simulink model "Main_v2"  (R2022b)
settings: Solver=ode23  StartTime=0.0  StopTime=sim_time-0.02
values from neighbouring files (symbols this model uses):
  bike_model = 1    [Main_sim.m]    (also in Startup_Script.m; Startup_Script_v2.m)
  bike_params = LoadBikeParameters(bike)    [Kalman_offline.m]    (also in Main_sim.m; Startup_Script.m; Startup_Script_v2.m; Startup_labview.m)
  C1 = [1 0 0 0 0 0 0 ... (first row only)    [Kalman_offline.m]    (also in Main_sim.m; Startup_Script.m; Startup_Script_v2.m; Startup_labview.m)
  counter = (Ts_GPS / Ts) - 1    (= 9)    [Kalman_offline.m]    (also in Main_sim.m; Startup_Script.m; Startup_Script_v2.m; Startup_labview.m)
  D_balancing_inner = 0    [Main_sim.m]    (also in Startup_Script.m; Startup_Script_v2.m; Startup_labview.m)
  D_balancing_outer = 0.0    (= 0)    [Main_sim.m]    (also in Startup_Script.m; Startup_Script_v2.m; Startup_labview.m)
  e1_max = abs(-k2*e2_max/k1)    [Main_sim.m]    (also in Startup_Script.m; Startup_Script_v2.m; Startup_labview.m)
  g = -9.81    [Kalman_offline.m]    (also in Main_sim.m = 9.81; Startup_Script.m = 9.81; Startup_Script_v2.m = 9.81; Startup_labview.m = 9.81)
  hor_dis = 10    [Main_sim.m]    (also in Startup_Script.m = 1; Startup_Script_v2.m = 1)
  I_balancing_inner = 0    [Main_sim.m]    (also in Startup_Script.m; Startup_Script_v2.m; Startup_labview.m)
  I_balancing_outer = 0.0    (= 0)    [Main_sim.m]    (also in Startup_Script.m; Startup_Script_v2.m; Startup_labview.m)
  initial_state_estimate = initial_state    [Main_sim.m]    (also in Startup_Script.m; Startup_Script_v2.m)
  k1 = K(1)    [Main_sim.m]    (also in Startup_Script.m; Startup_Script_v2.m; Startup_labview.m)
  k2 = K(2)    [Main_sim.m]    (also in Startup_Script.m; Startup_Script_v2.m; Startup_labview.m)
  Kalman_gain1 = Kalman_gain1'    [Kalman_offline.m]    (also in Main_sim.m; Startup_Script.m; Startup_Script_v2.m; Startup_labview.m)
  Kalman_gain2 = Kalman_gain2'    [Kalman_offline.m]    (also in Main_sim.m = Kalman_gain1(4:7,3:7); Startup_Script.m; Startup_Script_v2.m; Startup_labview.m = Kalman_gain1(4:7,3:7))
  linearized_sys = ss(A,B,C,D)    [Startup_Script_v2.m]
  P_balancing_inner = 3    [Main_sim.m]    (also in Startup_Script.m; Startup_Script_v2.m; Startup_labview.m = 1)
  P_balancing_outer = 1.3    [Main_sim.m]    (also in Startup_Script.m; Startup_Script_v2.m; Startup_labview.m = 1.75)
  Psiref = psiref'    [ReferenceGenerator.m]
  ref_dis = 0.01    [Main_sim.m]    (also in Startup_Script.m; Startup_Script_v2.m)
  ref_start_idx = 2    [Main_sim.m]    (also in Startup_Script.m; Startup_Script_v2.m)
  Ts = 0.01    [Kalman_offline.m]    (also in Main_sim.m; Startup_Script.m; Startup_Script_v2.m; Startup_labview.m)
  v = 3    [Main_sim.m]    (also in Startup_Script.m; Startup_Script_v2.m; Startup_labview.m = 2; Test_ss.m)
  Xref = xref'    [ReferenceGenerator.m]
  Yref = yref'    [ReferenceGenerator.m]
undefined symbols (not defined in the file or in its folder): initial_state, pert_deltadot_state, pert_deltadot_state_fun, pert_phidot_state, pert_phidot_state_fun
libraries: eeGeneralControl x3, slpidlib x2, simulink x2, cstblocks x1
(part 1 of 2)
settings Model: PauseTimes=0.16  Creator=Hadi Hajieghrary  LastModifiedBy=levi1
settings SolverCC: MaxConsecutiveMinStep=10  ZeroCrossAlgorithm=Adaptive  AlgebraicLoopSolver=TrustRegion  AutoInsertRateTranBlk=on
settings DebuggingCC: AlgebraicLoopMsg=none  UnconnectedInputMsg=warning  UnconnectedOutputMsg=warning  UnconnectedLineMsg=warning
settings ModelReferenceCC: EnableRefExpFcnMdlSchedulingChecks=on
settings RTWCC: DLArmComputeVersion=19.05

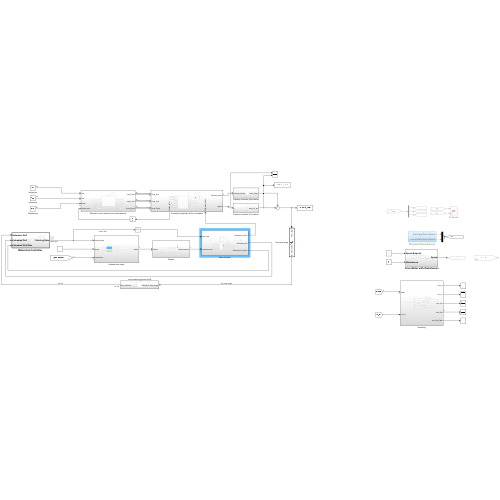
[thumbnail: Simulink's stored preview of the top-level diagram]
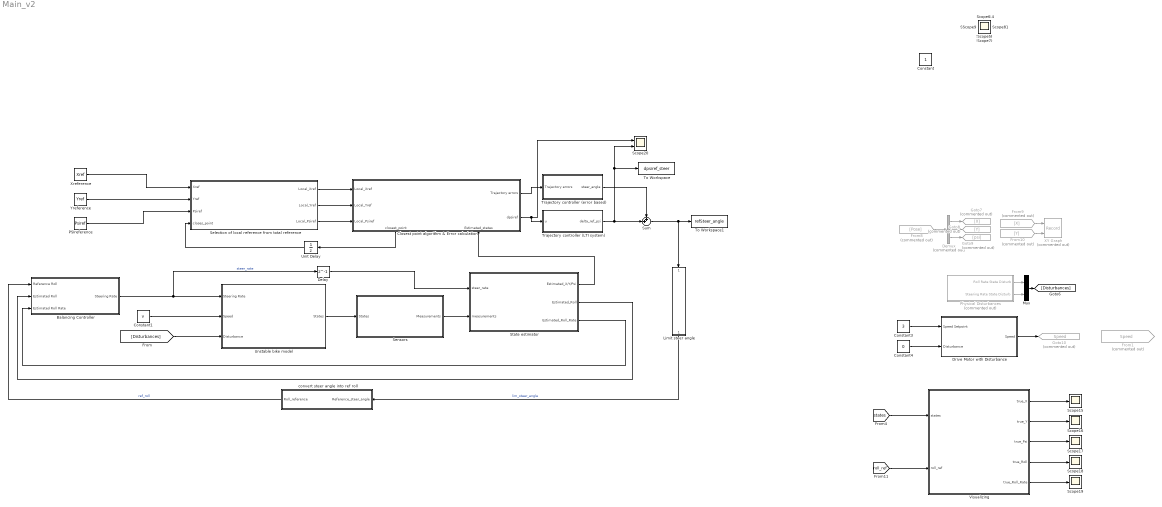
== system Main_v2 ==
  "Balancing Controller " : Subsystem  TreatAsAtomicUnit=on  SystemSampleTime=Ts
      settings: MinAlgLoopOccurrences=on
  Closest point algorithm & Error calculation : Subsystem
      settings: PortSchema="{\"entries\":[{\"content\":{\"sides\":[{\"content\":{\"connectorIds\":[\"In1\",\"In2\",\"In3\"]},\"type\":\"ConnectorPlacement.EquallySpacedRectSide\",\"uuid\":\"cc846df4-97c1-4e38-a551-63d96742d514\"},{\"content\":{\"connectorIds\":[\"Out1\",\"Out2\"],\"side\":\"RIGHT\"},\"type\":\"ConnectorPlacement.EquallySpacedRectSide\",\"uuid\":\"926eeee4-c51a-40d9-a9a1-df7a0c76cd55\"},{\"content\":{\"connectorIds\":[],\"side\":\"TOP\"},\"type\":\"ConnectorPlacement.EquallySpacedRectSide\",\"uuid\":\"e902e63c-5309-44b2-99e1-76b44c06d1f2\"},{\"content\":{\"connectorIds\":[\"Out3\",\"In4\"],\"side\":\"BOTTOM\"},\"type\":\"ConnectorPlacement.EquallySpacedRectSide\",\"uuid\":\"f92d60b4-b11f-4907-83c4-1907c5b6c496\"}]},\"type\":\"ConnectorPlacement.EquallySpacedConnector\",\"uuid\":\"17b67b4e-0a47-44a6-bf11-0cf8a9b1982c\"}],\"packageUris\":[\"http://schema.mathworks.com/mf0/Connector/R2020b\"],\"version\":\"1.0\"}"
  Constant1 : Constant  Value=v
  Constant3 : Constant  Value=3
  Constant4 : Constant  Value=0
  Delay : Delay  DelayLength=1  SampleTime=Ts
  Demux : Demux  Commented=on  Outputs=3
  Drive Motor with Disturbance : Subsystem
  From1 : From  Commented=on  GotoTag=Speed  TagVisibility=global
  From10 : From  Commented=on  GotoTag=Y
  From8 : From  Commented=on  GotoTag=Pose
  From9 : From  Commented=on  GotoTag=X
  Goto10 : Goto  Commented=on  GotoTag=Speed  TagVisibility=global
  Goto7 : Goto  Commented=on  GotoTag=X
  Goto8 : Goto  Commented=on  GotoTag=Y
  Goto9 : Goto  Commented=on  GotoTag=psi
  Limit steer angle : MATLAB Function  TreatAsAtomicUnit=on
  Mux : Mux  Inputs=2
  PSIreference : Constant  Value=Psiref
  Physical Disturbances : Subsystem  Commented=on
  Scope{,1..19} (20 alike) : Scope
  Scope20 : Scope  NumInputPorts=2
  Selection of local reference from total reference : Subsystem
  Sensors : Subsystem
  State estimator : Subsystem
  Sum : Sum  Inputs=++|
  To Workspace : ToWorkspace  VariableName=dpsiref_steer  SaveFormat=Timeseries  SampleTime=-1
  To Workspace1 : ToWorkspace  VariableName=refSteer_angle  SaveFormat=Timeseries  SampleTime=-1
  Trajectory controller (LTI system) : Subsystem
  Trajectory controller (error based) : Subsystem
  Unit Delay : UnitDelay  InitialCondition=ref_start_idx  SampleTime=Ts  HasFrameUpgradeWarning=on
  Unstable bike model : Subsystem
  Visualizing : Subsystem
  XY Graph : Record  Commented=on  FileSettingsInternal="{\"entries\":[{\"content\":{\"excelSettings\":{\"content\":{},\"type\":\"Streamout.ExcelSettings\"}},\"type\":\"Streamout.FileSettingStorage\",\"uuid\":\"82b19030-816e-4949-ae29-c4c1f1632771\"}],\"packageUris\":[\"http://schema.mathworks.com/mf0/streamout_blocks/R2020a\"],\"version\":\"1.0\"}"  Layout=[1 1]  SignalsInternal="{\"entries\":[{\"content\":{\"signals\":[]},\"type\":\"RecordBlkView.InputSignals\",\"uuid\":\"cc5346bf-f4f9-4ee2-bd9b-070395d24a3d\"}],\"packageUris\":[\"http://schema.mathworks.com/mf0/streamout_blocks/R2020a\"],\"version\":\"1.0\"}"  VisualizationBindings="{\"xyplotplugin\":{\"info\":[{\"series\":[],\"subplotID\":1}]}}"  CompatibilityTag=XY
  Xreference : Constant  Value=Xref
  Yreference : Constant  Value=Yref
  convert steer angle into ref roll : Subsystem
  Constant : Constant  IOType=siggen
  wires:
  From8/1 -> Demux/1
  Demux/1 -> Goto7/1
  Demux/2 -> Goto8/1
  Demux/3 -> Goto9/1
  From10/1 -> XY Graph/2
  From9/1 -> XY Graph/1
  Physical Disturbances/1(Roll Rate State Disturb) -> Mux/1
  Physical Disturbances/2(Steering Rate State Disturb) -> Mux/2
  Mux/1 -> [Disturbances]
  Drive Motor with Disturbance/1(Speed) -> Goto10/1
  Constant3/1 -> Drive Motor with Disturbance/1(Speed Setpoint)
  Constant4/1 -> Drive Motor with Disturbance/2(Disturbance)
  "Balancing Controller "/1(Steering Rate) -> Delay/1, Unstable bike model/1(Steering Rate)  "steer_rate"
  Selection of local reference from total reference/1(Local_Xref) -> Closest point algorithm & Error calculation/1(Local_Xref)
  Closest point algorithm & Error calculation/3(closest_point) -> Unit Delay/1
  Unit Delay/1 -> Selection of local reference from total reference/4(closes_point)
  Trajectory controller (error based)/1(steer_angle) -> Sum/1
  Closest point algorithm & Error calculation/2(dpsiref) -> Trajectory controller (LTI system)/1(u), Scope20/1
  Sum/1 -> Limit steer angle/1(steer_angle), To Workspace1/1
  Limit steer angle/1(lim_steer_angle) -> convert steer angle into ref roll/1(Reference_steer_angle)  "lim_steer_angle"
  convert steer angle into ref roll/1(Roll_reference) -> "Balancing Controller "/1(Reference Roll)  "ref_roll"
  [Disturbances] -> Unstable bike model/3(Disturbance)
  Sensors/1(Measurements) -> State estimator/2(measurements)
  Selection of local reference from total reference/2(Local_Yref) -> Closest point algorithm & Error calculation/2(Local_Yref)
  Selection of local reference from total reference/3(Local_Psiref) -> Closest point algorithm & Error calculation/3(Local_Psiref)
  [states] -> Visualizing/1(states)
  Visualizing/1(true_X) -> Scope15/1
  Visualizing/2(true_Y) -> Scope16/1
  Visualizing/3(true_Psi) -> Scope17/1
  Visualizing/4(true_Roll) -> Scope18/1
  Visualizing/5(true_Roll_Rate) -> Scope19/1
  [roll_ref] -> Visualizing/2(roll_ref)
  Unstable bike model/1(States) -> Sensors/1(States)
  Constant1/1 -> Unstable bike model/2(Speed)
  State estimator/2(Estimated_Roll) -> "Balancing Controller "/2(Estimated Roll)
  State estimator/3(Estimated_Roll_Rate) -> "Balancing Controller "/3(Estimated Roll Rate)
  Xreference/1 -> Selection of local reference from total reference/1(Xref)
  Yreference/1 -> Selection of local reference from total reference/2(Yref)
  PSIreference/1 -> Selection of local reference from total reference/3(Psiref)
  Delay/1 -> State estimator/1(steer_rate)
  State estimator/1(Estimated_X/Y/Psi) -> Closest point algorithm & Error calculation/4(Estimated_states)
  Closest point algorithm & Error calculation/1(Trajectory errors) -> Trajectory controller (error based)/1(Trajectory errors)
  Trajectory controller (LTI system)/1(delta_ref_psi) -> To Workspace/1, Scope20/2, Sum/2

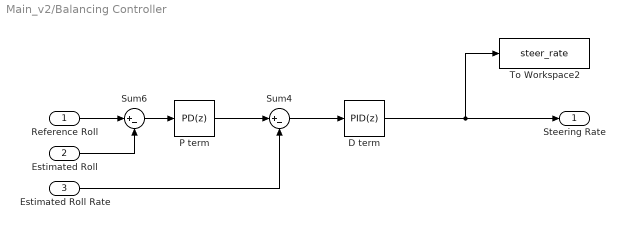
== system Main_v2/Balancing Controller  ==
  Reference Roll : Inport
  Estimated Roll : Inport  Port=2
  Estimated Roll Rate : Inport  Port=3
  D term : slpidlib/PID Controller  Controller=PID  Form=Parallel  TimeDomain=Discrete-time  UseExternalTs=off  SampleTime=Ts  IntegratorMethod=Forward Euler  FilterMethod=Forward Euler  ControllerParametersSource=internal  P=P_balancing_inner  I=I_balancing_inner  UseKiTs=off  D=D_balancing_inner  N=100  UseFilter=off  TunerSelectOption=Transfer Function Based (PID Tuner App)  InitialConditionSource=internal  InitialConditionForIntegrator=0  InitialConditionForFilter=0  DifferentiatorICPrevScaledInput=0  ExternalReset=none  TrackingMode=off  Kt=1  LimitOutput=off  SatLimitsSource=internal  UpperSaturationLimit=inf  LowerSaturationLimit=-inf  LinearizeAsGain=on  AntiWindupMode=none  Kb=1  LimitIntegrator=off  UpperIntegratorSaturationLimit=inf  LowerIntegratorSaturationLimit=-inf  POutMin=[]  POutMax=[]  IOutMin=[]  IOutMax=[]  DOutMin=[]  DOutMax=[]  NOutMin=[]  NOutMax=[]  SumOutMin=[]  SumOutMax=[]  SaturationOutMin=[]  SaturationOutMax=[]  PParamMin=[]  PParamMax=[]  IParamMin=[]  IParamMax=[]  DParamMin=[]  DParamMax=[]  NParamMin=[]  NParamMax=[]  KbParamMin=[]  KbParamMax=[]  KtParamMin=[]  KtParamMax=[]  KbOutMin=[]  KbOutMax=[]  KtOutMin=[]  KtOutMax=[]  IntegratorOutMin=[]  IntegratorOutMax=[]  FilterOutMin=[]  FilterOutMax=[]  SumI1OutMin=[]  SumI1OutMax=[]  SumI2OutMin=[]  SumI2OutMax=[]  SumI3OutMin=[]  SumI3OutMax=[]  SumI4OutMin=[]  SumI4OutMax=[]  SumDOutMin=[]  SumDOutMax=[]  DifferentiatorOutMin=[]  DifferentiatorOutMax=[]  FilterDiffOutCoefMin=[]  FilterDiffOutCoefMax=[]  ReciprocalOutMin=[]  ReciprocalOutMax=[]  SumDenOutMin=[]  SumDenOutMax=[]  SumNumOutMin=[]  SumNumOutMax=[]  DivideOutMin=[]  DivideOutMax=[]  UdiffTsProdOutMin=[]  UdiffTsProdOutMax=[]  NTsProdOutMin=[]  NTsProdOutMax=[]  UintegralTsProdOutMin=[]  UintegralTsProdOutMax=[]  UngainTsProdOutMin=[]  UngainTsProdOutMax=[]  IntegratorContinuousStateAttributes=''  IntegratorStateMustResolveToSignalObject=off  IntegratorRTWStateStorageClass=Auto  FilterContinuousStateAttributes=''  FilterStateMustResolveToSignalObject=off  FilterRTWStateStorageClass=Auto  ParallelPVariant=InternalParameters  IdealPVariant=Disabled  IVariant=InternalParameters  DVariant=InternalParameters  IntegratorVariant=Discrete  SatVariant=Disabled  AWVariant=Passthrough  PCopyVariant=Disabled  TRVariant=Disabled  FdbkBlocksVariant=Forward  IdealPFdbkVariant=Disabled  SatFdbkVariant=Disabled  DerivativeFilterVariant=Differentiator  NVariant=Passthrough  NCopyVariant=Disabled_SignalSpec  FilterICVariant=InternalICsDifferentiator  IntegratorICVariant=InternalICs  ExternalResetVariant=Disabled  TRSumVariant=Passthrough  SumFdbkVariant=Disabled  SumVariant=Sum_PID  TsampFilterVariant=InternalTs  TsampNgainVariant=Passthrough  TsampIntegralVariant=Passthrough  ExternalSaturationOutDataTypeStr=Inherit: Same as second input
  P term : slpidlib/PID Controller  Controller=PD  Form=Parallel  TimeDomain=Discrete-time  UseExternalTs=off  SampleTime=Ts  IntegratorMethod=Forward Euler  FilterMethod=Forward Euler  ControllerParametersSource=internal  P=P_balancing_outer  I=I_balancing_outer  UseKiTs=off  D=D_balancing_outer  N=100  UseFilter=off  TunerSelectOption=Transfer Function Based (PID Tuner App)  InitialConditionSource=internal  InitialConditionForIntegrator=0  InitialConditionForFilter=0  DifferentiatorICPrevScaledInput=0  ExternalReset=none  TrackingMode=off  Kt=1  LimitOutput=off  SatLimitsSource=internal  UpperSaturationLimit=inf  LowerSaturationLimit=-inf  LinearizeAsGain=on  AntiWindupMode=none  Kb=1  LimitIntegrator=off  UpperIntegratorSaturationLimit=inf  LowerIntegratorSaturationLimit=-inf  POutMin=[]  POutMax=[]  IOutMin=[]  IOutMax=[]  DOutMin=[]  DOutMax=[]  NOutMin=[]  NOutMax=[]  SumOutMin=[]  SumOutMax=[]  SaturationOutMin=[]  SaturationOutMax=[]  PParamMin=[]  PParamMax=[]  IParamMin=[]  IParamMax=[]  DParamMin=[]  DParamMax=[]  NParamMin=[]  NParamMax=[]  KbParamMin=[]  KbParamMax=[]  KtParamMin=[]  KtParamMax=[]  KbOutMin=[]  KbOutMax=[]  KtOutMin=[]  KtOutMax=[]  IntegratorOutMin=[]  IntegratorOutMax=[]  FilterOutMin=[]  FilterOutMax=[]  SumI1OutMin=[]  SumI1OutMax=[]  SumI2OutMin=[]  SumI2OutMax=[]  SumI3OutMin=[]  SumI3OutMax=[]  SumI4OutMin=[]  SumI4OutMax=[]  SumDOutMin=[]  SumDOutMax=[]  DifferentiatorOutMin=[]  DifferentiatorOutMax=[]  FilterDiffOutCoefMin=[]  FilterDiffOutCoefMax=[]  ReciprocalOutMin=[]  ReciprocalOutMax=[]  SumDenOutMin=[]  SumDenOutMax=[]  SumNumOutMin=[]  SumNumOutMax=[]  DivideOutMin=[]  DivideOutMax=[]  UdiffTsProdOutMin=[]  UdiffTsProdOutMax=[]  NTsProdOutMin=[]  NTsProdOutMax=[]  UintegralTsProdOutMin=[]  UintegralTsProdOutMax=[]  UngainTsProdOutMin=[]  UngainTsProdOutMax=[]  IntegratorContinuousStateAttributes=''  IntegratorStateMustResolveToSignalObject=off  IntegratorRTWStateStorageClass=Auto  FilterContinuousStateAttributes=''  FilterStateMustResolveToSignalObject=off  FilterRTWStateStorageClass=Auto  ParallelPVariant=InternalParameters  IdealPVariant=Disabled  IVariant=Disabled  DVariant=InternalParameters  IntegratorVariant=Disabled  SatVariant=Disabled  AWVariant=Disabled  PCopyVariant=Disabled  TRVariant=Disabled  FdbkBlocksVariant=Forward  IdealPFdbkVariant=Disabled  SatFdbkVariant=Disabled  DerivativeFilterVariant=Differentiator  NVariant=Passthrough  NCopyVariant=Disabled_SignalSpec  FilterICVariant=InternalICsDifferentiator  IntegratorICVariant=Disabled  ExternalResetVariant=Disabled  TRSumVariant=Passthrough  SumFdbkVariant=Disabled  SumVariant=Sum_PD  TsampFilterVariant=InternalTs  TsampNgainVariant=Passthrough  TsampIntegralVariant=Disabled_SignalSpec  ExternalSaturationOutDataTypeStr=Inherit: Same as second input
  Sum4 : Sum  Inputs=|+-
  Sum6 : Sum  Inputs=|+-
  To Workspace2 : ToWorkspace  VariableName=steer_rate  SaveFormat=Timeseries  SampleTime=-1
  Steering Rate : Outport
  wires:
  Sum4/1 -> D term/1
  Reference Roll/1 -> Sum6/1
  Sum6/1 -> P term/1
  Estimated Roll Rate/1 -> Sum4/2
  P term/1 -> Sum4/1
  D term/1 -> To Workspace2/1, Steering Rate/1
  Estimated Roll/1 -> Sum6/2

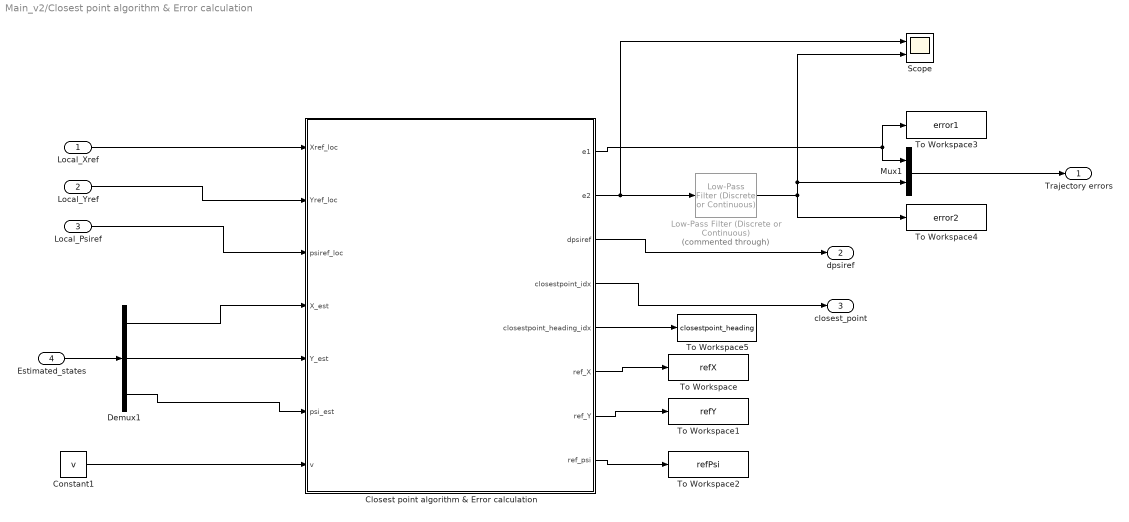
== system Main_v2/Closest point algorithm & Error calculation ==
  Local_Xref : Inport
  Local_Yref : Inport  Port=2
  Local_Psiref : Inport  Port=3
  Estimated_states : Inport  Port=4
  Closest point algorithm & Error calculation : MATLAB Function  TreatAsAtomicUnit=on
  Constant1 : Constant  Value=v
  Demux1 : Demux  Outputs=3
  Low-Pass Filter (Discrete or Continuous) : eeGeneralControl/Low-Pass Filter (Discrete or Continuous)  Commented=through  K=1  T=1  B=inf  A=-inf  init_option=Inherited from block input  x0=0  Ts=Ts
  Mux1 : Mux  Inputs=2
  Scope : Scope  NumInputPorts=2
  To Workspace : ToWorkspace  VariableName=refX  SaveFormat=Timeseries  SampleTime=-1
  To Workspace1 : ToWorkspace  VariableName=refY  SaveFormat=Timeseries  SampleTime=-1
  To Workspace2 : ToWorkspace  VariableName=refPsi  SaveFormat=Timeseries  SampleTime=-1
  To Workspace3 : ToWorkspace  VariableName=error1  SaveFormat=Timeseries  SampleTime=-1
  To Workspace4 : ToWorkspace  VariableName=error2  SaveFormat=Timeseries  SampleTime=-1
  To Workspace5 : ToWorkspace  VariableName=closestpoint_heading  SaveFormat=Timeseries  SampleTime=-1
  Trajectory errors : Outport
  dpsiref : Outport  Port=2
  closest_point : Outport  Port=3
  wires:
  Closest point algorithm & Error calculation/7(ref_Y) -> To Workspace1/1
  Constant1/1 -> Closest point algorithm & Error calculation/7(v)
  Closest point algorithm & Error calculation/8(ref_psi) -> To Workspace2/1
  Closest point algorithm & Error calculation/3(dpsiref) -> dpsiref/1
  Closest point algorithm & Error calculation/4(closestpoint_idx) -> closest_point/1
  Closest point algorithm & Error calculation/6(ref_X) -> To Workspace/1
  Demux1/2 -> Closest point algorithm & Error calculation/5(Y_est)
  Demux1/1 -> Closest point algorithm & Error calculation/4(X_est)
  Estimated_states/1 -> Demux1/1
  Local_Psiref/1 -> Closest point algorithm & Error calculation/3(psiref_loc)
  Local_Yref/1 -> Closest point algorithm & Error calculation/2(Yref_loc)
  Local_Xref/1 -> Closest point algorithm & Error calculation/1(Xref_loc)
  Closest point algorithm & Error calculation/1(e1) -> To Workspace3/1, Mux1/1
  Closest point algorithm & Error calculation/2(e2) -> Scope/1, Low-Pass Filter (Discrete or Continuous)/1
  Mux1/1 -> Trajectory errors/1
  Closest point algorithm & Error calculation/5(closestpoint_heading_idx) -> To Workspace5/1
  Low-Pass Filter (Discrete or Continuous)/1 -> Mux1/2, Scope/2, To Workspace4/1
  Demux1/3 -> Closest point algorithm & Error calculation/6(psi_est)

== system Main_v2/Drive Motor with Disturbance ==
  Speed Setpoint : Inport
  Disturbance : Inport  Port=2
  Sum2 : Sum  Inputs=++|
  Transfer Fcn : TransferFcn  Denominator=[2 1]
  Speed : Outport
  wires:
  Sum2/1 -> Speed/1
  Transfer Fcn/1 -> Sum2/2
  Speed Setpoint/1 -> Transfer Fcn/1
  Disturbance/1 -> Sum2/1

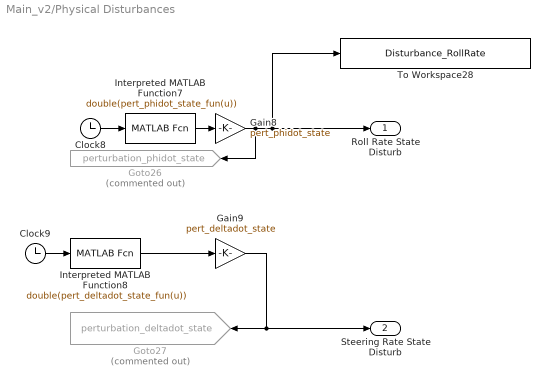
== system Main_v2/Physical Disturbances ==
  Clock8 : Clock
  Clock9 : Clock
  Gain8 : Gain  Gain=pert_phidot_state
  Gain9 : Gain  Gain=pert_deltadot_state
  Goto26 : Goto  Commented=on  GotoTag=perturbation_phidot_state  TagVisibility=global
  Goto27 : Goto  Commented=on  GotoTag=perturbation_deltadot_state  TagVisibility=global
  Interpreted MATLAB Function7 : MATLABFcn  MATLABFcn=double(pert_phidot_state_fun(u))
  Interpreted MATLAB Function8 : MATLABFcn  MATLABFcn=double(pert_deltadot_state_fun(u))
  To Workspace28 : ToWorkspace  VariableName=Disturbance_RollRate  SaveFormat=Timeseries  SampleTime=-1
  Roll Rate State Disturb : Outport
  Steering Rate State Disturb : Outport  Port=2
  wires:
  Interpreted MATLAB Function7/1 -> Gain8/1
  Clock8/1 -> Interpreted MATLAB Function7/1
  Gain8/1 -> Goto26/1, Roll Rate State Disturb/1, To Workspace28/1
  Interpreted MATLAB Function8/1 -> Gain9/1
  Clock9/1 -> Interpreted MATLAB Function8/1
  Gain9/1 -> Steering Rate State Disturb/1, Goto27/1

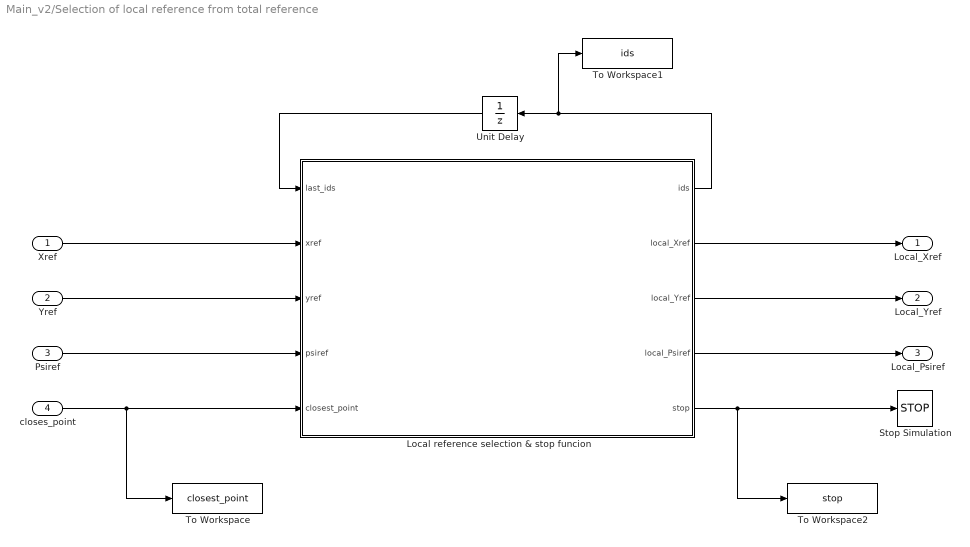
== system Main_v2/Selection of local reference from total reference ==
  Xref : Inport
  Yref : Inport  Port=2
  Psiref : Inport  Port=3
  closes_point : Inport  Port=4
  Local reference selection & stop funcion : MATLAB Function  TreatAsAtomicUnit=on
  Stop Simulation : Stop
  To Workspace : ToWorkspace  VariableName=closest_point  SaveFormat=Timeseries  SampleTime=-1
  To Workspace1 : ToWorkspace  VariableName=ids  SaveFormat=Timeseries  SampleTime=-1
  To Workspace2 : ToWorkspace  VariableName=stop  SaveFormat=Timeseries  SampleTime=-1
  Unit Delay : UnitDelay  InitialCondition=1  SampleTime=Ts  HasFrameUpgradeWarning=on
  Local_Xref : Outport
  Local_Yref : Outport  Port=2
  Local_Psiref : Outport  Port=3
  wires:
  Local reference selection & stop funcion/1(ids) -> To Workspace1/1, Unit Delay/1
  Unit Delay/1 -> Local reference selection & stop funcion/1(last_ids)
  closes_point/1 -> To Workspace/1, Local reference selection & stop funcion/5(closest_point)
  Xref/1 -> Local reference selection & stop funcion/2(xref)
  Yref/1 -> Local reference selection & stop funcion/3(yref)
  Psiref/1 -> Local reference selection & stop funcion/4(psiref)
  Local reference selection & stop funcion/5(stop) -> To Workspace2/1, Stop Simulation/1
  Local reference selection & stop funcion/2(local_Xref) -> Local_Xref/1
  Local reference selection & stop funcion/3(local_Yref) -> Local_Yref/1
  Local reference selection & stop funcion/4(local_Psiref) -> Local_Psiref/1

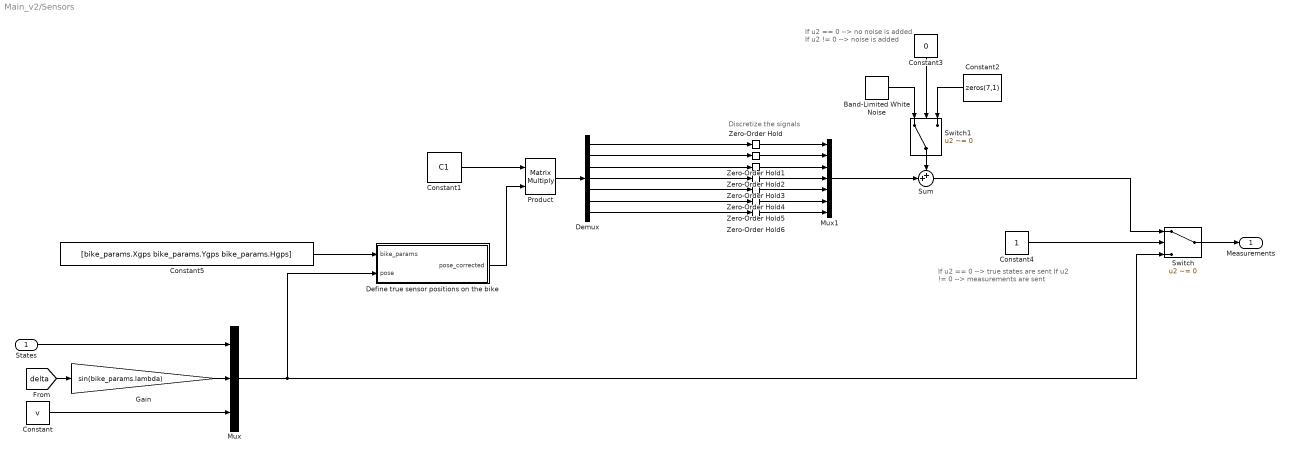
== system Main_v2/Sensors ==
  note: Discretize the signals
  note: If u2 == 0 --> no noise is added
      | If u2 != 0 --> noise is added
  note: If u2 == 0 --> true states are sent
      | If u2 != 0 --> measurements are sent
  States : Inport
  Band-Limited White Noise : simulink/Sources/Band-Limited White Noise  Cov=ones(7,1)*1e-3  Ts=Ts  seed=[23341]
  Constant : Constant  Value=v
  Constant1 : Constant  Value=C1
  Constant2 : Constant  Value=zeros(7,1)
  Constant3 : Constant  Value=0
  Constant4 : Constant
  Constant5 : Constant  Value=[bike_params.Xgps bike_params.Ygps bike_params.Hgps]
  Define true sensor positions on the bike : MATLAB Function  TreatAsAtomicUnit=on
  Demux : Demux  Outputs=7
  Gain : Gain  Gain=sin(bike_params.lambda)
  Mux : Mux  Inputs=3
  Mux1 : Mux  Inputs=7
  Product : Product  Multiplication=Matrix(*)
  Sum : Sum  Inputs=++|
  Switch : Switch  Criteria=u2 ~= 0  SaturateOnIntegerOverflow=off  InputSameDT=off
  Switch1 : Switch  Criteria=u2 ~= 0  SaturateOnIntegerOverflow=off  InputSameDT=off
  Zero-Order Hold : ZeroOrderHold  SampleTime=10*Ts
  Zero-Order Hold1 : ZeroOrderHold  SampleTime=10*Ts
  Zero-Order Hold{2..6} (5 alike) : ZeroOrderHold  SampleTime=Ts
  Measurements : Outport
  wires:
  [delta] -> Gain/1
  Constant/1 -> Mux/3
  Gain/1 -> Mux/2
  States/1 -> Mux/1
  Switch/1 -> Measurements/1
  Mux/1 -> Switch/3, Define true sensor positions on the bike/2(pose)
  Constant4/1 -> Switch/2
  Constant1/1 -> Product/1
  Switch1/1 -> Sum/1
  Band-Limited White Noise/1 -> Switch1/1
  Constant2/1 -> Switch1/3
  Constant3/1 -> Switch1/2
  Mux1/1 -> Sum/2
  Product/1 -> Demux/1
  Demux/2 -> Zero-Order Hold1/1
  Demux/3 -> Zero-Order Hold2/1
  Demux/4 -> Zero-Order Hold3/1
  Demux/5 -> Zero-Order Hold4/1
  Demux/6 -> Zero-Order Hold5/1
  Demux/7 -> Zero-Order Hold6/1
  Zero-Order Hold/1 -> Mux1/1
  Zero-Order Hold1/1 -> Mux1/2
  Zero-Order Hold2/1 -> Mux1/3
  Zero-Order Hold3/1 -> Mux1/4
  Zero-Order Hold4/1 -> Mux1/5
  Zero-Order Hold5/1 -> Mux1/6
  Zero-Order Hold6/1 -> Mux1/7
  Sum/1 -> Switch/1
  Demux/1 -> Zero-Order Hold/1
  Define true sensor positions on the bike/1(pose_corrected) -> Product/2
  Constant5/1 -> Define true sensor positions on the bike/1(bike_params)

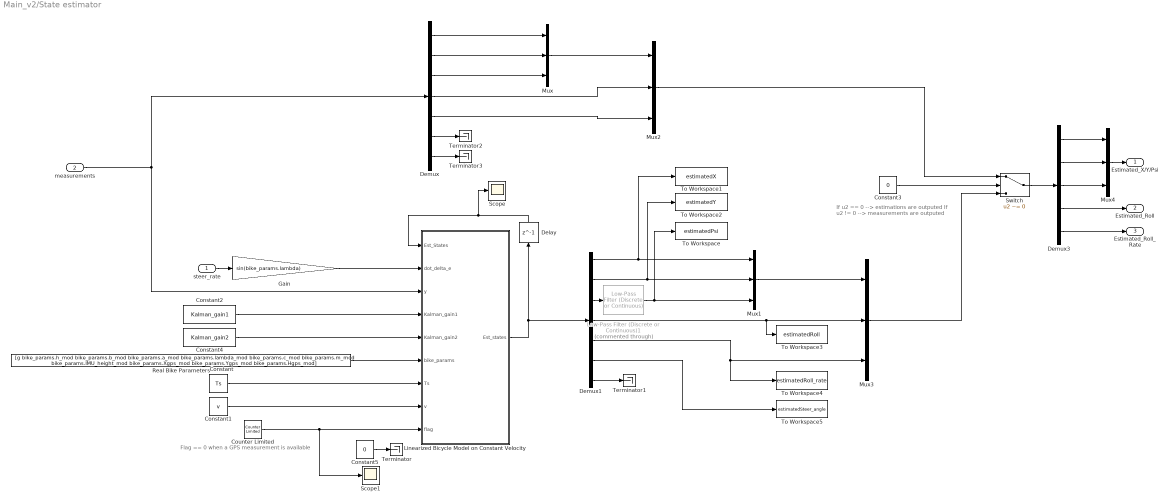
== system Main_v2/State estimator ==
  note: Flag == 0 when a GPS measurement is available
  note: If u2 == 0 --> estimations are outputed
      | If u2 != 0 --> measurements are outputed
  steer_rate : Inport
  measurements : Inport  Port=2
  Constant : Constant  Value=Ts
  Constant1 : Constant  Value=v
  Constant2 : Constant  Value=Kalman_gain1  SampleTime=Ts
  Constant3 : Constant  Value=0
  Constant4 : Constant  Value=Kalman_gain2  SampleTime=Ts
  Constant5 : Constant  Value=0
  Counter Limited : simulink/Sources/Counter Limited  uplimit=counter  tsamp=Ts
  Delay : Delay  DelayLength=1  InitialCondition=[initial_state_estimate.x initial_state_estimate.y initial_state_estimate.heading initial_state.roll initial_state.roll_rate initial_state.steering v]  SampleTime=Ts
  Demux : Demux  Outputs=7
  Demux1 : Demux  Outputs=7
  Demux3 : Demux  Outputs=5
  Gain : Gain  Gain=sin(bike_params.lambda)
  Linearized Bicycle Model on Constant Velocity : MATLAB Function  TreatAsAtomicUnit=on
  Low-Pass Filter (Discrete or Continuous)1 : eeGeneralControl/Low-Pass Filter (Discrete or Continuous)  Commented=through  K=1  T=1  B=inf  A=-inf  init_option=Inherited from block input  x0=0  Ts=Ts
  Mux{,1..4} (5 alike) : Mux  Inputs=3
  Real Bike Parameters : Constant  Value=[g bike_params.h_mod bike_params.b_mod bike_params.a_mod bike_params.lambda_mod bike_params.c_mod bike_params.m_mod bike_params.IMU_height_mod bike_params.Xgps_mod bike_params.Ygps_mod bike_params.Hgps_mod]  SampleTime=Ts
  Scope : Scope
  Scope1 : Scope
  Switch : Switch  Criteria=u2 ~= 0  SaturateOnIntegerOverflow=off  InputSameDT=off
  Terminator{,1..3} (4 alike) : Terminator
  To Workspace : ToWorkspace  VariableName=estimatedPsi  SaveFormat=Timeseries  SampleTime=-1
  To Workspace1 : ToWorkspace  VariableName=estimatedX  SaveFormat=Timeseries  SampleTime=-1
  To Workspace2 : ToWorkspace  VariableName=estimatedY  SaveFormat=Timeseries  SampleTime=-1
  To Workspace3 : ToWorkspace  VariableName=estimatedRoll  SaveFormat=Timeseries  SampleTime=-1
  To Workspace4 : ToWorkspace  VariableName=estimatedRoll_rate  SaveFormat=Timeseries  SampleTime=-1
  To Workspace5 : ToWorkspace  VariableName=estimatedSteer_angle  SaveFormat=Timeseries  SampleTime=-1
  Estimated_X/Y/Psi : Outport  VectorParamsAs1DForOutWhenUnconnected=off
  Estimated_Roll : Outport  Port=2  VectorParamsAs1DForOutWhenUnconnected=off
  Estimated_Roll_Rate : Outport  Port=3  VectorParamsAs1DForOutWhenUnconnected=off
  wires:
  Demux/3 -> Mux/3
  Linearized Bicycle Model on Constant Velocity/1(Est_states) -> Delay/1, Demux1/1
  Gain/1 -> Linearized Bicycle Model on Constant Velocity/2(dot_delta_e)
  Demux1/6 -> To Workspace5/1
  Constant/1 -> Linearized Bicycle Model on Constant Velocity/7(Ts)
  Demux1/5 -> Mux3/3, To Workspace4/1
  Delay/1 -> Scope/1, Linearized Bicycle Model on Constant Velocity/1(Est_States)
  steer_rate/1 -> Gain/1
  Real Bike Parameters/1 -> Linearized Bicycle Model on Constant Velocity/6(bike_params)
  Demux1/2 -> To Workspace2/1, Mux1/2
  measurements/1 -> Linearized Bicycle Model on Constant Velocity/3(y), Demux/1
  Demux/1 -> Mux/1
  Demux1/3 -> Low-Pass Filter (Discrete or Continuous)1/1
  Constant1/1 -> Linearized Bicycle Model on Constant Velocity/8(v)
  Demux1/1 -> Mux1/1, To Workspace1/1
  Demux/2 -> Mux/2
  Demux1/7 -> Terminator1/1
  Demux/7 -> Terminator3/1
  Demux/6 -> Terminator2/1
  Mux/1 -> Mux2/1
  Mux2/1 -> Switch/1
  Mux3/1 -> Switch/3
  Constant3/1 -> Switch/2
  Demux/4 -> Mux2/2
  Demux/5 -> Mux2/3
  Mux1/1 -> Mux3/1
  Demux1/4 -> To Workspace3/1, Mux3/2
  Switch/1 -> Demux3/1
  Demux3/1 -> Mux4/1
  Demux3/2 -> Mux4/2
  Demux3/3 -> Mux4/3
  Mux4/1 -> Estimated_X/Y/Psi/1
  Demux3/4 -> Estimated_Roll/1
  Demux3/5 -> Estimated_Roll_Rate/1
  Constant2/1 -> Linearized Bicycle Model on Constant Velocity/4(Kalman_gain1)
  Constant4/1 -> Linearized Bicycle Model on Constant Velocity/5(Kalman_gain2)
  Counter Limited/1 -> Scope1/1, Linearized Bicycle Model on Constant Velocity/9(flag)
  Low-Pass Filter (Discrete or Continuous)1/1 -> To Workspace/1, Mux1/3
  Constant5/1 -> Terminator/1

== system Main_v2/Trajectory controller (LTI system) ==
  u : Inport
  LTI System : cstblocks/LTI System  sys=tf(1,[bike_params.a/bike_params.b v/bike_params.b])  IC=[]
  MATLAB Function : MATLAB Function  Commented=on  TreatAsAtomicUnit=on
  Real Bike Parameters : Constant  Value=[ bike_params.b bike_params.a v]  SampleTime=Ts
  delta_ref_psi : Outport
  wires:
  u/1 -> MATLAB Function/1(dpsiref), LTI System/1
  Real Bike Parameters/1 -> MATLAB Function/2(bike_params)
  LTI System/1 -> delta_ref_psi/1

== system Main_v2/Trajectory controller (error based) ==
  Trajectory errors : Inport
  Constant : Constant  Value=k1
  Constant1 : Constant  Value=k2
  Constant2 : Constant  Value=e1_max
  Demux : Demux  Outputs=2
  Trajectory controller (Error based) : MATLAB Function  TreatAsAtomicUnit=on
  steer_angle : Outport
  wires:
  Trajectory errors/1 -> Demux/1
  Demux/1 -> Trajectory controller (Error based)/3(e1)
  Demux/2 -> Trajectory controller (Error based)/4(e2)
  Constant1/1 -> Trajectory controller (Error based)/2(k2)
  Constant/1 -> Trajectory controller (Error based)/1(k1)
  Constant2/1 -> Trajectory controller (Error based)/5(e1_max)
  Trajectory controller (Error based)/1(steer_angle) -> steer_angle/1

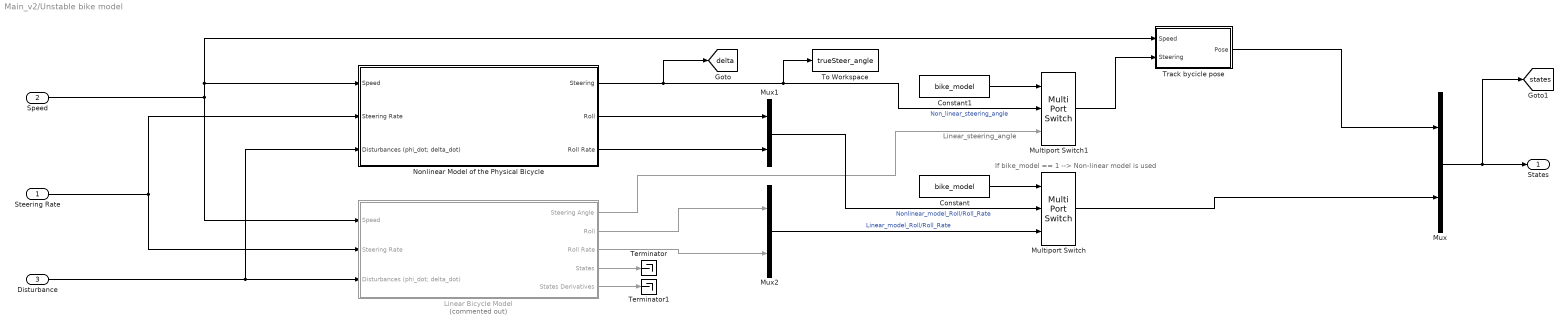
== system Main_v2/Unstable bike model ==
  note: If bike_model == 1 --> Non-linear model is used
  note: Linear_steering_angle
  Steering Rate : Inport
  Speed : Inport  Port=2
  Disturbance : Inport  Port=3
  Constant : Constant  Value=bike_model
  Constant1 : Constant  Value=bike_model
  Linear Bicycle Model : Subsystem  Commented=on  mask{Parameters=bike_params, linearized_sys=linearized_sys, Initial_State=initial_state}
      mask prompts: linearized_sys "Linearized System"; Initial_State "Initial State"
  Multiport Switch : MultiPortSwitch  Inputs=2  SaturateOnIntegerOverflow=off  InputSameDT=off
  Multiport Switch1 : MultiPortSwitch  Inputs=2  SaturateOnIntegerOverflow=off  InputSameDT=off
  Mux : Mux  Inputs=2
  Mux1 : Mux  Inputs=2
  Mux2 : Mux  Inputs=2
  Nonlinear Model of the Physical Bicycle : Subsystem  mask{Parameters=bike_params, Initial_State=initial_state}
      mask prompts: Initial_State "Initial State"
  Terminator : Terminator
  Terminator1 : Terminator
  To Workspace : ToWorkspace  VariableName=trueSteer_angle  SaveFormat=Timeseries  SampleTime=-1
  Track bycicle pose : Subsystem
  States : Outport
  tag scope: delta=global, states=global
  wires:
  Steering Rate/1 -> Linear Bicycle Model/2(Steering Rate), Nonlinear Model of the Physical Bicycle/2(Steering Rate)
  Constant/1 -> Multiport Switch/1
  Nonlinear Model of the Physical Bicycle/2(Roll) -> Mux1/1
  Nonlinear Model of the Physical Bicycle/3(Roll Rate) -> Mux1/2
  Nonlinear Model of the Physical Bicycle/1(Steering) -> [delta], To Workspace/1, Multiport Switch1/2  "Non_linear_steering_angle"
  Linear Bicycle Model/2(Roll) -> Mux2/1
  Linear Bicycle Model/3(Roll Rate) -> Mux2/2
  Linear Bicycle Model/1(Steering Angle) -> Multiport Switch1/3
  Mux1/1 -> Multiport Switch/2  "Nonlinear_model_Roll/Roll_Rate"
  Mux2/1 -> Multiport Switch/3  "Linear_model_Roll/Roll_Rate"
  Constant1/1 -> Multiport Switch1/1
  Mux/1 -> [states], States/1
  Multiport Switch/1 -> Mux/2
  Speed/1 -> Linear Bicycle Model/1(Speed), Track bycicle pose/1(Speed), Nonlinear Model of the Physical Bicycle/1(Speed)
  Disturbance/1 -> Nonlinear Model of the Physical Bicycle/3(Disturbances (phi_dot; delta_dot)), Linear Bicycle Model/3(Disturbances (phi_dot; delta_dot))
  Linear Bicycle Model/4(States) -> Terminator/1
  Linear Bicycle Model/5(States Derivatives) -> Terminator1/1
  Multiport Switch1/1 -> Track bycicle pose/2(Steering)
  Track bycicle pose/1(Pose) -> Mux/1

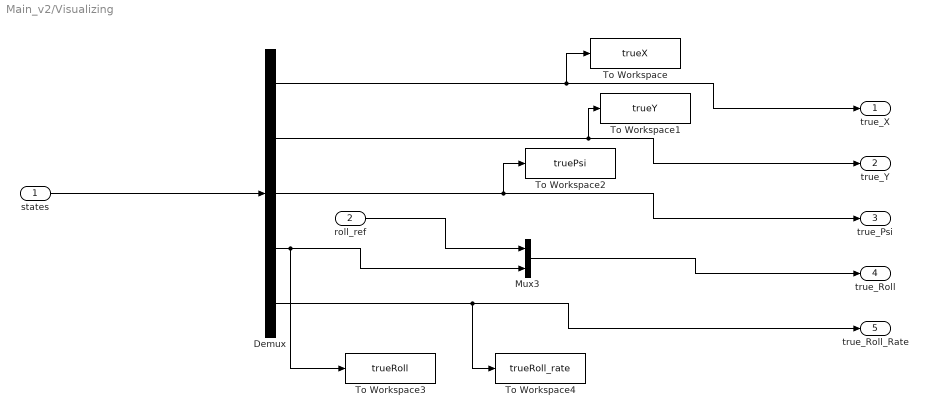
== system Main_v2/Visualizing ==
  states : Inport
  roll_ref : Inport  Port=2
  Demux : Demux  Outputs=5
  Mux3 : Mux  Inputs=2
  To Workspace : ToWorkspace  VariableName=trueX  SaveFormat=Timeseries  SampleTime=-1
  To Workspace1 : ToWorkspace  VariableName=trueY  SaveFormat=Timeseries  SampleTime=-1
  To Workspace2 : ToWorkspace  VariableName=truePsi  SaveFormat=Timeseries  SampleTime=-1
  To Workspace3 : ToWorkspace  VariableName=trueRoll  SaveFormat=Timeseries  SampleTime=-1
  To Workspace4 : ToWorkspace  VariableName=trueRoll_rate  SaveFormat=Timeseries  SampleTime=-1
  true_X : Outport
  true_Y : Outport  Port=2
  true_Psi : Outport  Port=3
  true_Roll : Outport  Port=4
  true_Roll_Rate : Outport  Port=5
  wires:
  states/1 -> Demux/1
  Demux/1 -> true_X/1, To Workspace/1
  Demux/3 -> To Workspace2/1, true_Psi/1
  roll_ref/1 -> Mux3/1
  Demux/4 -> To Workspace3/1, Mux3/2
  Mux3/1 -> true_Roll/1
  Demux/5 -> To Workspace4/1, true_Roll_Rate/1
  Demux/2 -> To Workspace1/1, true_Y/1

== system Main_v2/convert steer angle into ref roll ==
  Reference_steer_angle : Inport
  Constant : Constant  Value=[bike_params.lambda bike_params.b g]
  Constant5 : Constant  Value=v
  Convert steer angle to roll : MATLAB Function  TreatAsAtomicUnit=on
  To Workspace : ToWorkspace  VariableName=refRoll  SaveFormat=Timeseries  SampleTime=-1
  Roll_reference : Outport
  tag scope: roll_ref=global
  wires:
  Reference_steer_angle/1 -> Convert steer angle to roll/1(steer_angle_ref)
  Constant/1 -> Convert steer angle to roll/2(bike_params)
  Constant5/1 -> Convert steer angle to roll/3(v)
  Convert steer angle to roll/1(roll_ref) -> To Workspace/1, Roll_reference/1, [roll_ref]

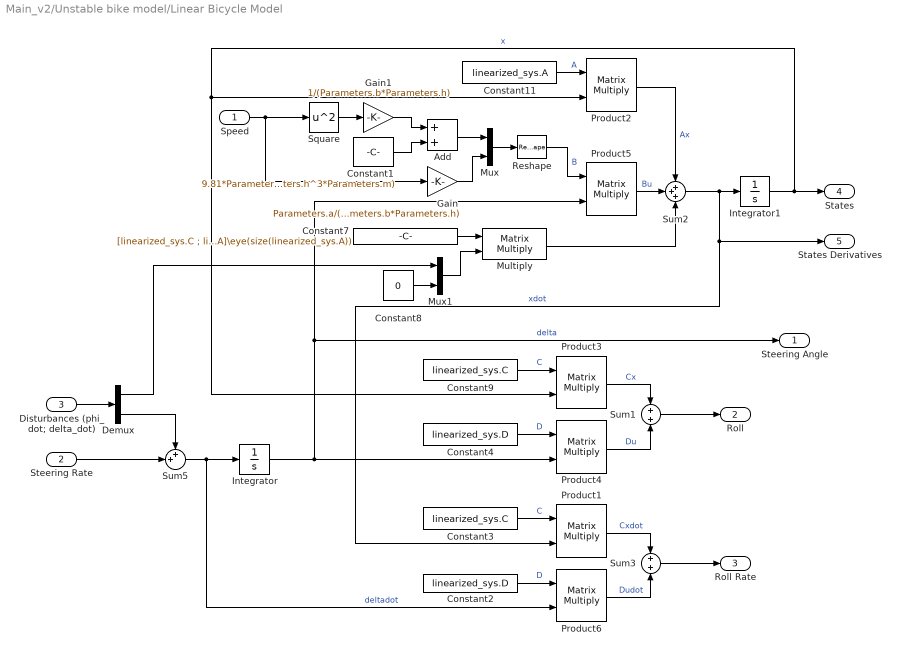
== system Main_v2/Unstable bike model/Linear Bicycle Model ==
  Speed : Inport
  Steering Rate : Inport  Port=2
  Disturbances (phi_dot; delta_dot) : Inport  Port=3
  Add : Sum
  Constant1 : Constant  Value=9.81*Parameters.inertia_front/(Parameters.h^3*Parameters.m)
  Constant11 : Constant  Value=linearized_sys.A  VectorParams1D=off
  Constant2 : Constant  Value=linearized_sys.D  VectorParams1D=off
  Constant3 : Constant  Value=linearized_sys.C  VectorParams1D=off
  Constant4 : Constant  Value=linearized_sys.D  VectorParams1D=off
  Constant7 : Constant  Value=[linearized_sys.C ; linearized_sys.C*linearized_sys.A]\eye(size(linearized_sys.A))  VectorParams1D=off
  Constant8 : Constant  Value=0
  Constant9 : Constant  Value=linearized_sys.C  VectorParams1D=off
  Demux : Demux  Outputs=2
  Gain : Gain  Gain=Parameters.a/(Parameters.b*Parameters.h)
  Gain1 : Gain  Gain=1/(Parameters.b*Parameters.h)
  Integrator : Integrator  InitialCondition=Initial_State.steering
  Integrator1 : Integrator  InitialCondition=[linearized_sys.C ; linearized_sys.C*linearized_sys.A]\[Initial_State.roll ; Initial_State.roll_rate]
  Multiply : Product  Multiplication=Matrix(*)
  Mux : Mux  Inputs=2
  Mux1 : Mux  Inputs=2
  Product{1..6} (6 alike) : Product  SCDEnableBlockLinearizationSpecification=on  Multiplication=Matrix(*)
  Reshape : Reshape  OutputDimensionality=Customize  OutputDimensions=[size(linearized_sys.B,1),size(linearized_sys.B,2)]
  Square : Math  Operator=square  SignedPower=on
  Sum1 : Sum
  Sum2 : Sum  Inputs=+++
  Sum3 : Sum
  Sum5 : Sum  Inputs=++|
  Steering Angle : Outport  VectorParamsAs1DForOutWhenUnconnected=off
  Roll : Outport  Port=2  VectorParamsAs1DForOutWhenUnconnected=off
  Roll Rate : Outport  Port=3  VectorParamsAs1DForOutWhenUnconnected=off
  States : Outport  Port=4  VectorParamsAs1DForOutWhenUnconnected=off
  States Derivatives : Outport  Port=5  VectorParamsAs1DForOutWhenUnconnected=off
  wires:
  Product5/1 -> Sum2/2  "Bu"
  Constant11/1 -> Product2/1  "A"
  Sum2/1 -> Product1/2, States Derivatives/1, Integrator1/1  "xdot"
  Product2/1 -> Sum2/1  "Ax"
  Sum1/1 -> Roll/1
  Reshape/1 -> Product5/1  "B"
  Steering Rate/1 -> Sum5/2
  Product4/1 -> Sum1/2  "Du"
  Product3/1 -> Sum1/1  "Cx"
  Gain1/1 -> Add/1
  Constant1/1 -> Add/2
  Mux/1 -> Reshape/1
  Add/1 -> Mux/1
  Gain/1 -> Mux/2
  Speed/1 -> Square/1, Gain/1
  Square/1 -> Gain1/1
  Disturbances (phi_dot; delta_dot)/1 -> Demux/1
  Sum5/1 -> Integrator/1, Product6/2  "deltadot"
  Multiply/1 -> Sum2/3
  Demux/1 -> Mux1/1
  Constant7/1 -> Multiply/1
  Mux1/1 -> Multiply/2
  Constant8/1 -> Mux1/2
  Demux/2 -> Sum5/1
  Constant9/1 -> Product3/1  "C"
  Constant4/1 -> Product4/1  "D"
  Sum3/1 -> Roll Rate/1
  Integrator1/1 -> States/1, Product2/2, Product3/2  "x"
  Product6/1 -> Sum3/2  "Dudot"
  Constant3/1 -> Product1/1  "C"
  Product1/1 -> Sum3/1  "Cxdot"
  Constant2/1 -> Product6/1  "D"
  Integrator/1 -> Product5/2, Steering Angle/1, Product4/2  "delta"

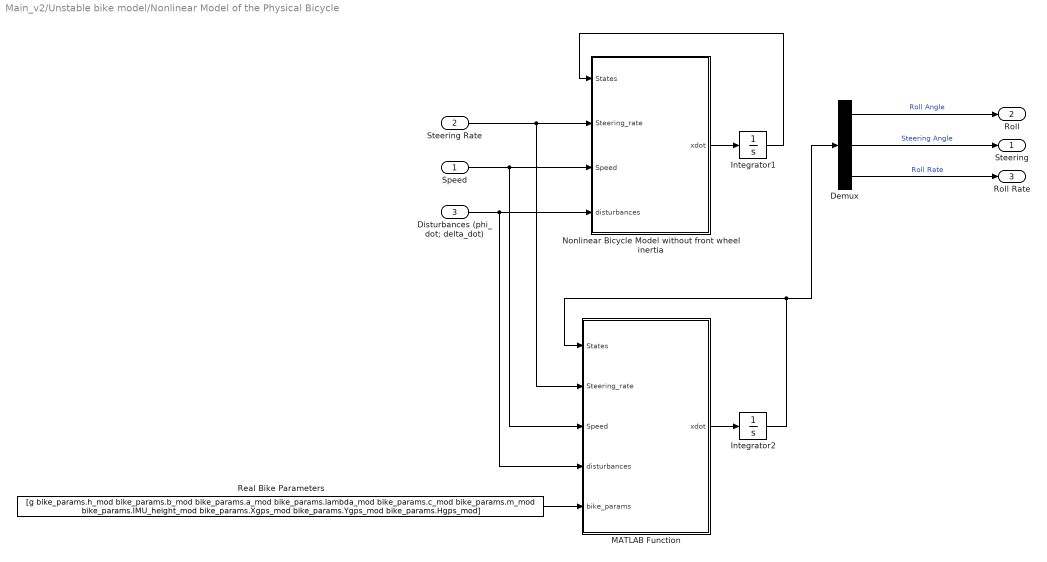
== system Main_v2/Unstable bike model/Nonlinear Model of the Physical Bicycle ==
  Speed : Inport
  Steering Rate : Inport  Port=2
  Disturbances (phi_dot; delta_dot) : Inport  Port=3
  Demux : Demux  Outputs=3
  Integrator1 : Integrator  InitialCondition=[Initial_State.roll ; Initial_State.steering ; Initial_State.roll_rate]
  Integrator2 : Integrator  InitialCondition=[Initial_State.roll ; Initial_State.steering ; Initial_State.roll_rate]
  MATLAB Function : MATLAB Function  TreatAsAtomicUnit=on
  Nonlinear Bicycle Model without front wheel inertia : MATLAB Function  TreatAsAtomicUnit=on  mask{Parameters=Parameters}
  Real Bike Parameters : Constant  Value=[g bike_params.h_mod bike_params.b_mod bike_params.a_mod bike_params.lambda_mod bike_params.c_mod bike_params.m_mod bike_params.IMU_height_mod bike_params.Xgps_mod bike_params.Ygps_mod bike_params.Hgps_mod]  SampleTime=Ts
  Steering : Outport  VectorParamsAs1DForOutWhenUnconnected=off
  Roll : Outport  Port=2  VectorParamsAs1DForOutWhenUnconnected=off
  Roll Rate : Outport  Port=3  VectorParamsAs1DForOutWhenUnconnected=off
  wires:
  Integrator1/1 -> Nonlinear Bicycle Model without front wheel inertia/1(States)
  Demux/1 -> Roll/1  "Roll Angle"
  Nonlinear Bicycle Model without front wheel inertia/1(xdot) -> Integrator1/1
  Speed/1 -> MATLAB Function/3(Speed), Nonlinear Bicycle Model without front wheel inertia/3(Speed)
  Demux/3 -> Roll Rate/1  "Roll Rate"
  Demux/2 -> Steering/1  "Steering Angle"
  Steering Rate/1 -> MATLAB Function/2(Steering_rate), Nonlinear Bicycle Model without front wheel inertia/2(Steering_rate)
  Disturbances (phi_dot; delta_dot)/1 -> MATLAB Function/4(disturbances), Nonlinear Bicycle Model without front wheel inertia/4(disturbances)
  Real Bike Parameters/1 -> MATLAB Function/5(bike_params)
  MATLAB Function/1(xdot) -> Integrator2/1
  Integrator2/1 -> MATLAB Function/1(States), Demux/1

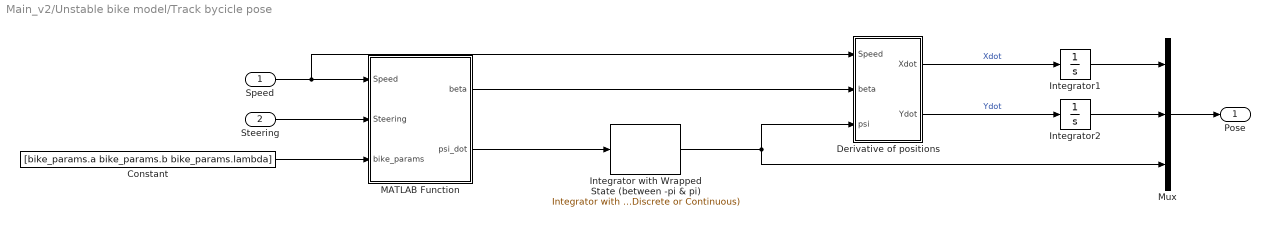
== system Main_v2/Unstable bike model/Track bycicle pose ==
  Speed : Inport
  Steering : Inport  Port=2
  Constant : Constant  Value=[bike_params.a bike_params.b bike_params.lambda]
  Derivative of positions : MATLAB Function  TreatAsAtomicUnit=on
  Integrator with Wrapped State (between -pi & pi) : eeGeneralControl/Integrator with Wrapped State (Discrete or Continuous)  LabelModeActiveChoice=Discrete  WrappedStateUpperValue=pi  WrappedStateLowerValue=-pi  x0=initial_state.heading  Ts=Ts
  Integrator1 : Integrator  InitialCondition=initial_state.x
  Integrator2 : Integrator  InitialCondition=initial_state.y
  MATLAB Function : MATLAB Function  TreatAsAtomicUnit=on
  Mux : Mux  Inputs=3
  Pose : Outport
  wires:
  Derivative of positions/2(Ydot) -> Integrator2/1  "Ydot"
  Steering/1 -> MATLAB Function/2(Steering)
  Integrator2/1 -> Mux/2
  Mux/1 -> Pose/1
  Derivative of positions/1(Xdot) -> Integrator1/1  "Xdot"
  Speed/1 -> MATLAB Function/1(Speed), Derivative of positions/1(Speed)
  Integrator1/1 -> Mux/1
  MATLAB Function/1(beta) -> Derivative of positions/2(beta)
  Constant/1 -> MATLAB Function/3(bike_params)
  MATLAB Function/2(psi_dot) -> Integrator with Wrapped State (between -pi & pi)/1
  Integrator with Wrapped State (between -pi & pi)/1 -> Derivative of positions/3(psi), Mux/3

== matlab function Main_v2/Selection of local reference from total reference/Local reference selection & stop funcion ==
  data: last_ids input; ids output; xref input; local_Xref output size=Nn [..30000]; local_Yref output size=Nn [..30000]; local_Psiref output size=Nn [..30000]; yref input; psiref input; closest_point input; ref_dis parameter; hor_dis parameter; stop output
function [ids,local_Xref,local_Yref,local_Psiref,stop] = fcn(last_ids,xref,yref,psiref,closest_point, ref_dis, hor_dis)
% Local reference trajectory starts at point before the current closest
% point and has a length of M
ids=last_ids+closest_point-1;      % calculate the initial index of the points that will be sent to next block (first point of local_ref)

Ns=ceil(hor_dis/ref_dis);          % Th,Ts is definited in "StudentProject2021.m", Ns is the number of points sent to next block
M=ids+Ns;                          % calculate the end index of the end index that will be sent to next block
n=size(xref,1);                    % size of whole trajectory points 
if M>n                             % if reached near end of reference, local trajectry becomes shorter
    M=n;
end

% Temporary simulation STOP to prevent singularity error once approaching
% the end of the trajectory
% Simulation stops before the end of the reference trajectory
stop = 0;
if ids>=n-ceil(n/10)
    stop = 1;
end

% Start always at second value of total reference
% if ids == 1
% ids = 2;
% end

% Select local reference from total reference
local_Xref=xref(ids-1:M,1);
local_Yref=yref(ids-1:M,1);
local_Psiref=psiref(ids-1:M,1);

== matlab function Main_v2/Limit steer angle ==
  data: steer_angle input; lim_steer_angle output
function lim_steer_angle= fcn(steer_angle)

% limit steer angle between -pi/4 and pi/4
if steer_angle>=pi/4
    steer_angle=pi/4;
end

if steer_angle<=-pi/4
    steer_angle=-pi/4;
   
end
lim_steer_angle = steer_angle;

== matlab function Main_v2/Trajectory controller (LTI system)/MATLAB Function ==
  data: dpsiref input; delta_ref_psi output; bike_params input
function delta_ref_psi = fcn(dpsiref, bike_params)
a = bike_params(1);
b = bike_params(2);
v = bike_params(3);

%Calculate the contribution in reference steering angle from deltapsi
delta_ref_psi = tf(1,[a/b v/b])*dpsiref;
end
